simulink model "Permocar_sim_with_torque"  (R2018a)
settings: Solver=VariableStepAuto  StartTime=0.0  StopTime=50  FixedStep=0.001  MaxStep=0.001  RelTol=1e-10
values from neighbouring files (symbols this model uses):
  Ad = SYSd.A    [Permocar_luenberger.m]
  B1 = SYScr.B(1,2)    [d2c_motors.m]
  B2 = SYScl.B(1,2)    [d2c_motors.m]
  Bd = SYSd.B    [Permocar_luenberger.m]
  Cd = SYSd.C    [Permocar_luenberger.m]
  K1 = SYScr.A(1,1)    [d2c_motors.m]
  K2 = SYScr.B(1,1)    [d2c_motors.m]
  K3 = SYScl.A(1,1)    [d2c_motors.m]
  K4 = SYScl.B(1,1)    [d2c_motors.m]
  Lk = place(SYSd.A',SYSd.C',[Pvd;Pwd])'    [Permocar_luenberger.m]
  Ts = 0.05    [system_setup.m]
  Ts_kf = 0.01    [system_setup.m]
  V1 = 1/(m+(2*Iw/R^2))    (= 0.00625969994827)    [system_setup.m]
  V2 = -mc*d    (= -25)    [system_setup.m]
  VT = 1/R    (= 6.06060606061)    [system_setup.m]
  W1 = 1/(I + ((2*Iw*L^2)/R^2))    (= 0.0683212405443)    [system_setup.m]
  W2 = V2    (= -25)    [system_setup.m]
  WT = L/R    (= 1.72727272727)    [system_setup.m]
undefined symbols (not defined in the file or in its folder): DiscIntNeverNeededParam
libraries: simulink x2
settings Model: Creator=olov  LastModifiedBy=olov
settings RTWCC: Toolchain=Catkin  TargetLang=C++
settings GRTTargetCC: TargetLangStandard=C++03 (ISO)  MultiInstanceERTCode=on  CodeInterfacePackaging=C++ class

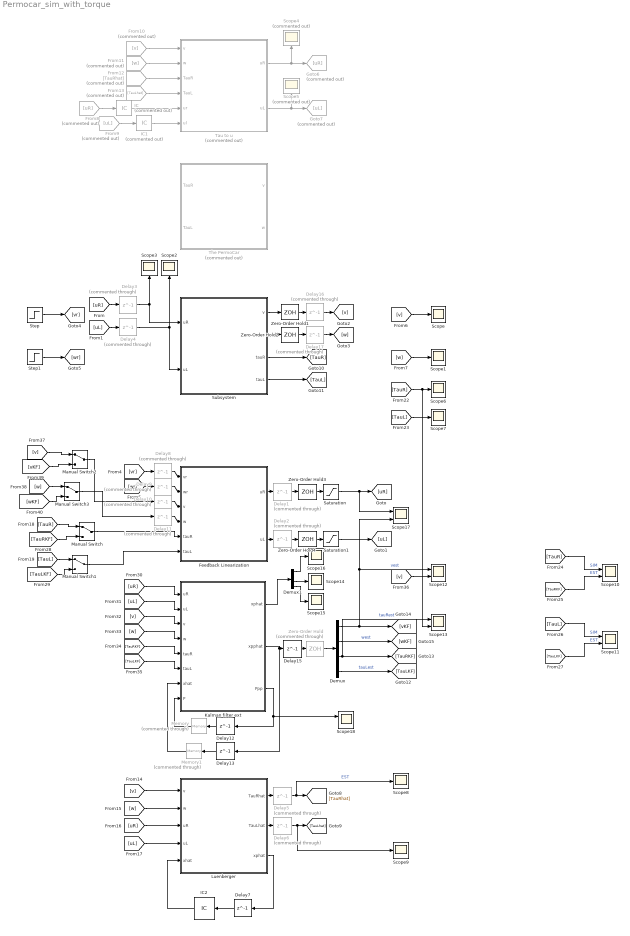
== system Permocar_sim_with_torque ==
  Delay{1..6,8..11,16..17} (12 alike) : Delay  Commented=through  DelayLength=1  InitialCondition=0  SampleTime=Ts
  Delay12 : Delay  DelayLength=1  InitialCondition=0  SampleTime=Ts_kf
  Delay13 : Delay  DelayLength=1  InitialCondition=[0;0;0;0]  SampleTime=Ts_kf
  Delay15 : Delay  DelayLength=1  InitialCondition=0  SampleTime=Ts_kf
  Delay7 : Delay  DelayLength=1  InitialCondition=0  SampleTime=Ts
  Demux : Demux
  Demux1 : Demux
  Feedback Linearization : MATLAB Function  TreatAsAtomicUnit=on
  From10 : From  Commented=on  GotoTag=v
  From11 : From  Commented=on  GotoTag=w
  From12 : From  Commented=on  GotoTag=TauRhat
  From13 : From  Commented=on  GotoTag=TauLhat
  From8 : From  Commented=on  GotoTag=uR
  From9 : From  Commented=on  GotoTag=uL
  Goto6 : Goto  Commented=on  GotoTag=uR
  Goto7 : Goto  Commented=on  GotoTag=uL
  IC : InitialCondition  Commented=on  Value=0
  IC1 : InitialCondition  Commented=on  Value=0
  IC2 : InitialCondition  Value=[0;0;0;0]
  Kalman filter ext : MATLAB Function  TreatAsAtomicUnit=on
  Luenberger : MATLAB Function  TreatAsAtomicUnit=on
  Manual Switch{,1..3} (4 alike) : ManualSwitch
  Memory : Memory  Commented=through
  Memory1 : Memory  Commented=through
  Saturation : Saturate  UpperLimit=1  LowerLimit=-1
  Saturation1 : Saturate  UpperLimit=1  LowerLimit=-1
  Scope{,1..3,6..9,14..16} (11 alike) : Scope
  Scope{10..13,17..18} (6 alike) : Scope  NumInputPorts=2
  Scope4 : Scope  Commented=on
  Scope5 : Scope  Commented=on
  Step : Step  Time=15  SampleTime=0
  Step1 : Step  Time=30  After=0  SampleTime=0
  Subsystem : Subsystem
  Tau to u : MATLAB Function  Commented=on  TreatAsAtomicUnit=on
  The PermoCar : Subsystem  Commented=on
  Zero-Order Hold : ZeroOrderHold  Commented=through  SampleTime=Ts_kf
  Zero-Order Hold1 : ZeroOrderHold  SampleTime=Ts
  Zero-Order Hold2 : ZeroOrderHold  SampleTime=Ts
  Zero-Order Hold3 : ZeroOrderHold  SampleTime=Ts_kf
  Zero-Order Hold4 : ZeroOrderHold  SampleTime=Ts_kf
  wires:
  Manual Switch3/1 -> Delay11/1
  Manual Switch2/1 -> Delay10/1
  [vr] -> Delay8/1
  [wr] -> Delay9/1
  Step/1 -> [vr]
  Step1/1 -> [wr]
  [w] -> Scope1/1
  Subsystem/1(v) -> Zero-Order Hold1/1
  Subsystem/2(w) -> Zero-Order Hold2/1
  [uL] -> Delay4/1
  [uR] -> Delay3/1
  IC/1 -> Tau to u/5(ur)
  IC1/1 -> Tau to u/6(ul)
  Tau to u/1(uR) -> Scope4/1, Goto6/1
  Tau to u/2(uL) -> Scope5/1, Goto7/1
  From8/1 -> IC/1
  From9/1 -> IC1/1
  From10/1 -> Tau to u/1(v)
  From11/1 -> Tau to u/2(w)
  From12/1 -> Tau to u/3(TauR)
  From13/1 -> Tau to u/4(TauL)
  Delay3/1 -> Scope3/1, Subsystem/1(uR)
  Delay4/1 -> Scope2/1, Subsystem/2(uL)
  [v] -> Luenberger/1(v)
  [w] -> Luenberger/2(w)
  [uR] -> Luenberger/3(uR)
  [uL] -> Luenberger/4(uL)
  Manual Switch/1 -> Feedback Linearization/5(tauR)
  Manual Switch1/1 -> Feedback Linearization/6(tauL)
  IC2/1 -> Luenberger/5(xhat)
  Luenberger/3(xphat) -> Delay7/1
  Delay7/1 -> IC2/1
  Feedback Linearization/1(uR) -> Delay1/1
  Delay1/1 -> Zero-Order Hold3/1
  Feedback Linearization/2(uL) -> Delay2/1
  Delay2/1 -> Zero-Order Hold4/1
  Subsystem/3(tauR) -> [TauR]
  Subsystem/4(tauL) -> [TauL]
  [TauR] -> Scope13/2, Scope6/1
  [TauL] -> Scope7/1
  Delay5/1 -> Scope8/1, [TauRhat]  "EST"
  Luenberger/1(TauRhat) -> Delay5/1
  Luenberger/2(TauLhat) -> Delay6/1
  Delay6/1 -> Scope9/1, [TauLhat]
  [TauR] -> Scope10/1  "SIM"
  [TauRKF] -> Scope10/2  "EST"
  [TauL] -> Scope11/1  "SIM"
  [TauLKF] -> Scope11/2  "EST"
  [TauR] -> Manual Switch/1
  [TauRKF] -> Manual Switch/2
  [TauL] -> Manual Switch1/1
  [TauLKF] -> Manual Switch1/2
  Delay9/1 -> Feedback Linearization/2(wr)
  Delay10/1 -> Feedback Linearization/3(v)
  Delay11/1 -> Feedback Linearization/4(w)
  Delay8/1 -> Feedback Linearization/1(vr)
  Kalman filter ext/3(Ppp) -> Scope18/1, Delay12/1
  Delay12/1 -> Memory/1
  Kalman filter ext/2(xpphat) -> Delay15/1, Delay13/1
  Delay13/1 -> Memory1/1
  [uR] -> Kalman filter ext/1(uR)
  [uL] -> Kalman filter ext/2(uL)
  [v] -> Kalman filter ext/3(v)
  [w] -> Kalman filter ext/4(w)
  [TauRKF] -> Kalman filter ext/5(tauR)
  [TauLKF] -> Kalman filter ext/6(tauL)
  Demux/1 -> Scope17/2, Scope12/1, [vKF]  "vest"
  Demux/3 -> Scope13/1, [TauRKF]  "tauRest"
  Demux/4 -> [TauLKF]  "tauLest"
  [v] -> Scope12/2
  Kalman filter ext/1(xphat) -> Demux1/1
  Demux1/3 -> Scope14/1
  Memory/1 -> Kalman filter ext/8(P)
  Memory1/1 -> Kalman filter ext/7(xhat)
  Demux1/4 -> Scope15/1
  Demux1/1 -> Scope16/1
  Delay16/1 -> [v]
  Delay17/1 -> [w]
  Saturation/1 -> Scope17/1, [uR]
  Saturation1/1 -> [uL]
  Delay15/1 -> Zero-Order Hold/1
  Demux/2 -> [wKF]  "west"
  [w] -> Manual Switch3/1
  [v] -> Manual Switch2/1
  [vKF] -> Manual Switch2/2
  [wKF] -> Manual Switch3/2
  Zero-Order Hold/1 -> Demux/1
  Zero-Order Hold1/1 -> Delay16/1
  Zero-Order Hold2/1 -> Delay17/1
  [v] -> Scope/1
  Zero-Order Hold3/1 -> Saturation/1
  Zero-Order Hold4/1 -> Saturation1/1

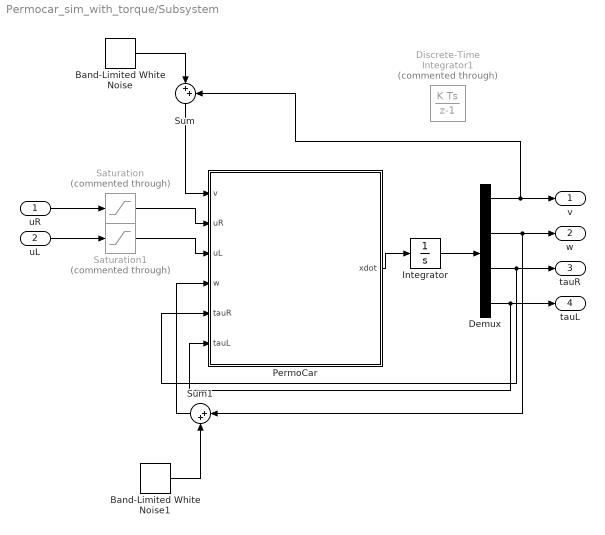
== system Permocar_sim_with_torque/Subsystem ==
  uR : Inport
  uL : Inport  Port=2
  Band-Limited White Noise : simulink/Sources/Band-Limited White Noise  Cov=[0]  Ts=Ts  seed=[23341]
  Band-Limited White Noise1 : simulink/Sources/Band-Limited White Noise  Cov=[0]  Ts=Ts  seed=[23341]
  Demux : Demux
  Discrete-Time Integrator1 : DiscreteIntegrator  Commented=through  SampleTime=0.05  ICPrevOutput=DiscIntNeverNeededParam  ICPrevScaledInput=DiscIntNeverNeededParam
  Integrator : Integrator
  PermoCar : MATLAB Function  TreatAsAtomicUnit=on
  Saturation : Saturate  Commented=through  UpperLimit=1  LowerLimit=-1
  Saturation1 : Saturate  Commented=through  UpperLimit=1  LowerLimit=-1
  Sum : Sum  Inputs=|++
  Sum1 : Sum  Inputs=|++
  v : Outport
  w : Outport  Port=2
  tauR : Outport  Port=3
  tauL : Outport  Port=4
  wires:
  uL/1 -> Saturation1/1
  uR/1 -> Saturation/1
  Demux/1 -> Sum/2, v/1
  Demux/2 -> Sum1/1, w/1
  PermoCar/1(xdot) -> Integrator/1
  Integrator/1 -> Demux/1
  Demux/3 -> PermoCar/5(tauR), tauR/1
  Demux/4 -> PermoCar/6(tauL), tauL/1
  Sum/1 -> PermoCar/1(v)
  Band-Limited White Noise/1 -> Sum/1
  Band-Limited White Noise1/1 -> Sum1/2
  Sum1/1 -> PermoCar/4(w)
  Saturation/1 -> PermoCar/2(uR)
  Saturation1/1 -> PermoCar/3(uL)

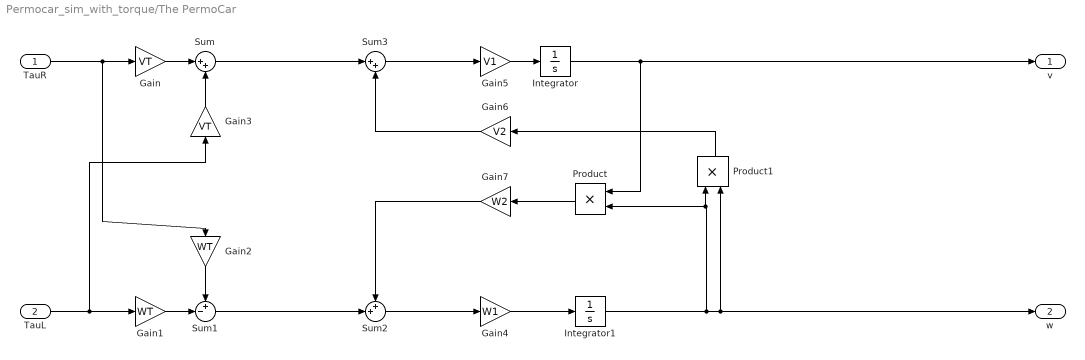
== system Permocar_sim_with_torque/The PermoCar ==
  TauR : Inport
  TauL : Inport  Port=2
  Gain : Gain  Gain=VT
  Gain1 : Gain  Gain=WT
  Gain2 : Gain  Gain=WT
  Gain3 : Gain  Gain=VT
  Gain4 : Gain  Gain=W1
  Gain5 : Gain  Gain=V1
  Gain6 : Gain  Gain=V2
  Gain7 : Gain  Gain=W2
  Integrator : Integrator
  Integrator1 : Integrator
  Product : Product
  Product1 : Product
  Sum : Sum  Inputs=|++
  Sum1 : Sum  Inputs=+-|
  Sum2 : Sum  Inputs=++|
  Sum3 : Sum  Inputs=|++
  v : Outport
  w : Outport  Port=2
  wires:
  TauL/1 -> Gain3/1, Gain1/1
  TauR/1 -> Gain2/1, Gain/1
  Sum/1 -> Sum3/1
  Sum1/1 -> Sum2/2
  Sum2/1 -> Gain4/1
  Sum3/1 -> Gain5/1
  Gain4/1 -> Integrator1/1
  Gain5/1 -> Integrator/1
  Product1/1 -> Gain6/1
  Gain6/1 -> Sum3/2
  Product/1 -> Gain7/1
  Gain7/1 -> Sum2/1
  Integrator/1 -> Product/1, v/1
  Integrator1/1 -> Product1/2, w/1, Product1/1, Product/2
  Gain/1 -> Sum/1
  Gain3/1 -> Sum/2
  Gain1/1 -> Sum1/2
  Gain2/1 -> Sum1/1

== matlab function Permocar_sim_with_torque/Subsystem/PermoCar ==
  data: xdot output; v input; uR input; uL input; w input; tauR input; tauL input; Ts parameter; K1 parameter; K2 parameter; K3 parameter; K4 parameter; B1 parameter; B2 parameter
function xdot = fcn(v,uR,uL ,w, tauR, tauL,Ts,K1, K2, K3, K4, B1, B2)

xdot = [0 0 0 0]';

u = [uR;uL];

K1 = K1*1;
K2 = K2*1;
K3 = K3*1;
K4 = K4*1;
B1 = B1*0;
B2 = B2*0;

mc = 100;
mw = 7.5;
m = mc + 2*mw;

R = 0.165;
L = 0.285;
d = 0.25;

Ic = ((1/2)*mc*d^2);
Im = (mw*(R^2));
Iw = (mw*L^2);

I = (Ic + mc*d^2 + 2*mw*L^2 + 2*Im);



A1 = (-mc*d)/(m + 2*Iw/(R^2));
A2 = (1/(R*(m + 2*Iw/(R^2))));
A3 = (1/(R*(m + 2*Iw/(R^2))));
A4 = (mc*d)/(I + (2*Iw*L^2)/(R^2));
A5 = L/(R*((I + (2*Iw*L^2)/(R^2))));
A6 = -L/(R*((I + (2*Iw*L^2)/(R^2))));

%     
f = [A1*w^2 + A2*tauR + A3*tauL;       
         A4*w*v + A5*tauR + A6*tauL;
            K1*tauR + K2*(L*w + v);
                 K3*tauL + K4*(v - L*w)];

g = [0 0;
         0 0;
            B1 0;
               0 B2];         

    
xdot = f + g*u;

== matlab function Permocar_sim_with_torque/Feedback Linearization ==
  data: vr input; wr input; uR output; v input; w input; uL output; tauR input; tauL input; Ts parameter; K1 parameter; K2 parameter; K3 parameter; K4 parameter; B1 parameter; B2 parameter
function [uR,uL] = fcn(vr,wr, v,w, tauR, tauL,Ts,K1, K2, K3, K4, B1, B2)

uR = 0;
uL = 0;

r = [vr;
        wr];

mc = 100;
mw = 7.5;
m = mc + 2*mw;

R = 0.165;
L = 0.285;
d = 0.25;

Ic = (1/2)*mc*d^2;
Im = mw*(R^2);
Iw = mw*L^2;

I = Ic + mc*d^2 + 2*mw*L^2 + 2*Im;

ksi = 1;
Trsv = 4;
wnv = 3.8/(ksi*Trsv);

ksi = 1;
Trsw = 4;
wnw = 3.8/(ksi*Trsw);
% 
% LL = [wnv^2 2*ksi*wnv 0 0;
%         0 0 wnw^2 2*ksi*wnw]

K11 = wnv^2;
K12 = 2*ksi*wnv;
K13 = 0;
K14 = 0;
K21 = 0;
K22 = 0;
K23 = wnw^2;
K24 = 2*ksi*wnw;

Kr11 = wnv^2;
Kr12 = 0;
Kr21 = 0;
Kr22 = wnw^2;


uK = [- ((m*R^2 + 2*Iw)*(K11*v - Kr11*vr + K13*w - Kr12*wr + (R*(K1*tauR + K2*v + K2*L*w))/(m*R^2 + 2*Iw) + (R*(K3*tauL + K4*v - K4*L*w))/(m*R^2 + 2*Iw) + (K14*R*(L*tauR - L*tauL + R*d*mc*v*w))/(2*Iw*L^2 + I*R^2) + (K12*R*(- R*d*mc*w^2 + tauL + tauR))/(m*R^2 + 2*Iw) - (2*R^3*d*mc*w*(L*tauR - L*tauL + R*d*mc*v*w))/((2*Iw*L^2 + I*R^2)*(m*R^2 + 2*Iw))))/(2*B1*R) - ((2*Iw*L^2 + I*R^2)*(K21*v - Kr21*vr + K23*w - Kr22*wr + (L*R*(K1*tauR + K2*v + K2*L*w))/(2*Iw*L^2 + I*R^2) - (L*R*(K3*tauL + K4*v - K4*L*w))/(2*Iw*L^2 + I*R^2) + (K24*R*(L*tauR - L*tauL + R*d*mc*v*w))/(2*Iw*L^2 + I*R^2) + (K22*R*(- R*d*mc*w^2 + tauL + tauR))/(m*R^2 + 2*Iw) + (R^3*d*mc*v*(L*tauR - L*tauL + R*d*mc*v*w))/(2*Iw*L^2 + I*R^2)^2 + (R^3*d*mc*w*(- R*d*mc*w^2 + tauL + tauR))/((2*Iw*L^2 + I*R^2)*(m*R^2 + 2*Iw))))/(2*B1*L*R);
   ((2*Iw*L^2 + I*R^2)*(K21*v - Kr21*vr + K23*w - Kr22*wr + (L*R*(K1*tauR + K2*v + K2*L*w))/(2*Iw*L^2 + I*R^2) - (L*R*(K3*tauL + K4*v - K4*L*w))/(2*Iw*L^2 + I*R^2) + (K24*R*(L*tauR - L*tauL + R*d*mc*v*w))/(2*Iw*L^2 + I*R^2) + (K22*R*(- R*d*mc*w^2 + tauL + tauR))/(m*R^2 + 2*Iw) + (R^3*d*mc*v*(L*tauR - L*tauL + R*d*mc*v*w))/(2*Iw*L^2 + I*R^2)^2 + (R^3*d*mc*w*(- R*d*mc*w^2 + tauL + tauR))/((2*Iw*L^2 + I*R^2)*(m*R^2 + 2*Iw))))/(2*B2*L*R) - ((m*R^2 + 2*Iw)*(K11*v - Kr11*vr + K13*w - Kr12*wr + (R*(K1*tauR + K2*v + K2*L*w))/(m*R^2 + 2*Iw) + (R*(K3*tauL + K4*v - K4*L*w))/(m*R^2 + 2*Iw) + (K14*R*(L*tauR - L*tauL + R*d*mc*v*w))/(2*Iw*L^2 + I*R^2) + (K12*R*(- R*d*mc*w^2 + tauL + tauR))/(m*R^2 + 2*Iw) - (2*R^3*d*mc*w*(L*tauR - L*tauL + R*d*mc*v*w))/((2*Iw*L^2 + I*R^2)*(m*R^2 + 2*Iw))))/(2*B2*R)];
 
uR = uK(1);
uL = uK(2);

== matlab function Permocar_sim_with_torque/Tau to u ==
  data: v input; w input; uR output; TauR input; TauL input; uL output; ur input; ul input
function [uR,uL] = fcn(v, w, TauR, TauL,ur, ul)

L = 0.285;
R = 0.165;
m = 115;

uR = 0;
uL = 0;

vr = L*w + v;
vl = v - L*w;

Thetar = [10.95, 13.52, 0.83];
Thetal = [9.61, 11.45, 0.85];

inputr = [TauR/(R*m), vr, ur]';
inputl = [TauL/(R*m), vl, ul]';
        
uR = Thetar*inputr;
uL = Thetal*inputl;

== matlab function Permocar_sim_with_torque/Luenberger ==
  data: v input; w input; uR input; uL input; TauRhat output; TauLhat output; Ad parameter; Lk parameter; xhat input; xphat output; Cd parameter; Bd parameter
function [TauRhat,TauLhat, xphat] = fcn(v,w,uR, uL, Ad ,Lk, xhat, Cd, Bd)

TauRhat = 0;
TauLhat = 0;

y = [v; w];
u = [uR;uL];

xphat = Ad*xhat + Lk*(y - Cd*xhat) + Bd*u;


TauRhat = xhat(3);
TauLhat = xhat(4);

== matlab function Permocar_sim_with_torque/Kalman filter ext ==
  data: xphat output; uR input; uL input; xpphat output; v input; w input; Ppp output; tauR input; tauL input; xhat input; P input; Ts_kf parameter; K1 parameter; K2 parameter; B2 parameter; K3 parameter; K4 parameter; B1 parameter
function [xphat,xpphat,Ppp] = fcn(uR,uL, v,w, tauR, tauL,xhat,P,Ts_kf,K1, K2, B2, K3, K4, B1)


xpphat = [0;0;0;0];
xphat = [0;0;0;0];
Ppp = zeros(4,4);

u = [uR;
        uL];

x = [v;
        w;
            tauR;
                tauL];

v=xhat(1);
w=xhat(2);
tauR=xhat(3);
tauL=xhat(4);

mc = 100;
mw = 7.5;
m = mc + 2*mw;

R = 0.165;
L = 0.285;
d = 0.25;

Ic = (1/2)*mc*d^2;
Im = mw*(R^2);
Iw = mw*L^2;

I = Ic + mc*d^2 + 2*mw*L^2 + 2*Im;


A1 = (-mc*d)/(m + 2*Iw/(R^2));
A2 = (1/(R*(m + 2*Iw/(R^2))));
A3 = (1/(R*(m + 2*Iw/(R^2))));
A4 = (mc*d)/(I + (2*Iw*L^2)/(R^2));
A5 = L/(R*((I + (2*Iw*L^2)/(R^2))));
A6 = -L/(R*((I + (2*Iw*L^2)/(R^2))));

Ak = [0, -(2*d*mc*w)/(m + (2*Iw)/R^2), 1/(R*(m + (2*Iw)/R^2)), 1/(R*(m + (2*Iw)/R^2));
    (d*mc*w)/(I + (2*Iw*L^2)/R^2), (d*mc*v)/(I + (2*Iw*L^2)/R^2), L/(R*(I + (2*Iw*L^2)/R^2)), -L/(R*(I + (2*Iw*L^2)/R^2));
    K2, K2*L, K1, 0;
    K4, -K4*L, 0, K3];

Ak=(eye(4)+Ts_kf*Ak);

Bk = [0 0;
         0 0;
            B1 0;
               0 B2]*Ts_kf;
           
 Ck = [1 0 0 0;
         0 1 0 0];
%Ck = eye(4);    
    
y = Ck*x;    
    
Dk = [0 0;
        0 0;];
    
    
Nk = 10*[1 0 0 0;
            0 1 0 0;
                0 0 1 0;
                    0 0 0 1];
Qk = [1 0 0 0;
        0 1 0 0;
            0 0 1 0;
                0 0 0 1];
 Rk = [100 0;
         0 100];
            
% Rk = [0 0 0 0;
%        0 0 0 0;
%            0 0 0.01 0;
%                0 0 0 0.01];


    
xphat = Ak*xhat + Bk*u;
Pp = Ak*P*Ak' + Nk*Qk*Nk';

Kk = Pp*Ck'*inv(Ck*Pp*Ck' + Rk);
ytilde = y - Ck*xphat;
xpphat = xphat + Kk*ytilde;
Ppp = Pp - Kk*Ck*Pp;
